simulink model "CommandeAModeleInterne"  (R2017a)
settings: Solver=VariableStepAuto  StartTime=0.0  StopTime=100  RelTol=1e-3
settings Model: Creator=Iheb  LastModifiedBy=PC

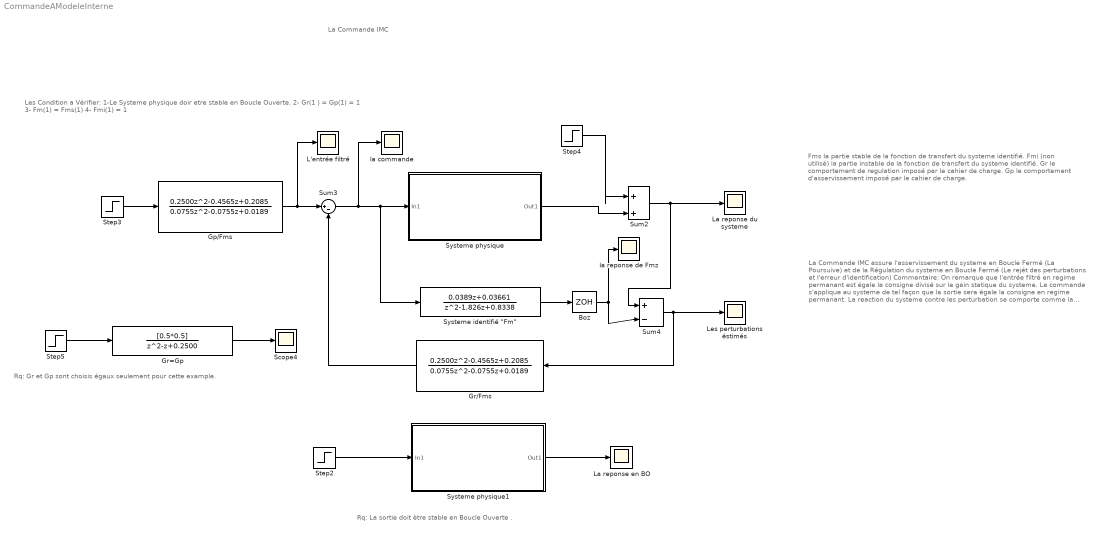
== system CommandeAModeleInterne ==
  note: Rq: Gr et Gp sont choisis égaux seulement pour cette example.
  note: La Commande IMC
  note: Fms la partie stable de la fonction de transfert du systeme identifié.
      | Fmi (non utilisé) la partie instable de la fonction de transfert du systeme identifié.
      | Gr le comportement de regulation imposé par le cahier de charge.
      | Gp le comportement d'asservissement imposé par le cahier de charge.
  note: Les Condition a Vérifier:
      | 1-Le Systeme physique doir etre stable en Boucle Ouverte.
      | 2- Gr(1 ) = Gp(1) = 1
      | 3- Fm(1) = Fms(1)
      | 4- Fmi(1) = 1
  note: La Commande IMC assure l'asservissement du systeme en Boucle Fermé (La Poursuive) et de la Régulation du systeme en Boucle Fermé (Le rejét des perturbations et l'erreur d'identification)
      |
      | Commentaire:
      | On remarque que l'entrée filtré en regime permanant est égale la consigne divisé sur le gain statique du systeme.
      | La commande s'applique au systeme de tel façon que la sortie sera égale la consigne en regime permanant.
      | La reaction du systeme contre les perturbation se comporte comme la reaction de la fonction Gr et la meme chose pour la poursuive.(Gr et Gp represente le cahier de charge pour notre systeme)
  note: Rq: La sortie doit ètre stable en Boucle Ouverte .
  "Boz " : ZeroOrderHold
  Gp/Fms : DiscreteTransferFcn  Numerator="[0.2500   -0.4565    0.2085]"  Denominator="[0.0755   -0.0755    0.0189]"
  "Gr/Fms " : DiscreteTransferFcn  Numerator="[0.2500   -0.4565    0.2085]"  Denominator="[0.0755   -0.0755    0.0189]"
  Gr=Gp : DiscreteTransferFcn  Numerator=[0.5*0.5]  Denominator="[1.0000   -1.0000    0.2500]"
  L'entrée filtré : Scope
  "La reponse du systeme " : Scope
  "La reponse en BO " : Scope
  Les perturbations éstimés : Scope
  Scope4 : Scope
  Step2 : Step  Time=0  SampleTime=0
  Step3 : Step  Time=0  SampleTime=0
  Step4 : Step  Time=50  SampleTime=0
  Step5 : Step  Time=0  SampleTime=0
  Sum2 : Sum  Inputs=|++
  Sum3 : Sum  Inputs=|+-
  Sum4 : Sum  Inputs=|+-
  "Systeme identifié \"Fm\"" : DiscreteTransferFcn  Numerator=[0.0389 0.03661]  Denominator=[1 -1.826 0.8338]
  Systeme physique : Subsystem
  Systeme physique1 : Subsystem
  "la commande " : Scope
  la reponse de Fmz : Scope
  wires:
  Sum2/1 -> Sum4/1, "La reponse du systeme "/1
  Step4/1 -> Sum2/1
  "Systeme identifié \"Fm\""/1 -> "Boz "/1
  Step3/1 -> Gp/Fms/1
  "Boz "/1 -> Sum4/2, la reponse de Fmz/1
  Sum4/1 -> "Gr/Fms "/1, Les perturbations éstimés/1
  Gp/Fms/1 -> L'entrée filtré/1, Sum3/1
  Gr=Gp/1 -> Scope4/1
  Step5/1 -> Gr=Gp/1
  "Gr/Fms "/1 -> Sum3/2
  Sum3/1 -> "la commande "/1, Systeme physique/1(In1), "Systeme identifié \"Fm\""/1
  Systeme physique/1(Out1) -> Sum2/2
  Step2/1 -> Systeme physique1/1(In1)
  Systeme physique1/1(Out1) -> "La reponse en BO "/1

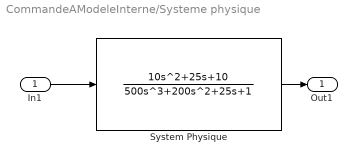
== system CommandeAModeleInterne/Systeme physique ==
  In1 : Inport
  System Physique : TransferFcn  Numerator=[10 25 10]  Denominator=[500 200 25 1]
  Out1 : Outport
  wires:
  In1/1 -> System Physique/1
  System Physique/1 -> Out1/1

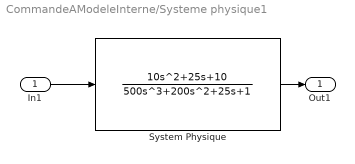
== system CommandeAModeleInterne/Systeme physique1 ==
  In1 : Inport
  System Physique : TransferFcn  Numerator=[10 25 10]  Denominator=[500 200 25 1]
  Out1 : Outport
  wires:
  System Physique/1 -> Out1/1
  In1/1 -> System Physique/1
